simulink model "SF051A_SnsrOffsLrng"  (R2013b)
settings: Solver=FixedStepDiscrete  SolverMode=SingleTasking  StartTime=0.0  StopTime=1  FixedStep=0.002  RelTol=1e-3
undefined symbols (not defined in the file): ARCHGLBPRM_10MILLISEC_SEC_F32, ARCHGLBPRM_2MILLISEC_SEC_F32, ARCHGLBPRM_2PI_ULS_F32, ARCHGLBPRM_FLOATZEROTHD_ULS_F32, ARCHGLBPRM_PIOVER180_ULS_F32, CNV100MICROSECTOMILLISEC_MILLISECPERCNT_F32, CNV100MICROSECTOSEC_SECPERCNT_F32, COVRAMTRXNIT_ULS_F32, HWAUTHYTHD_ULS_F32, HWTQLRNGSTSLRND_CNT_U08, HWTQLRNGSTSNEGOFFS_CNT_U08, HWTQLRNGSTSNOTLRND_CNT_U08, HWTQLRNGSTSPOSOFFS_CNT_U08, HWTQLRNGSTSZEROOFFS_CNT_U08, HWTQLRNGTMRHILIM_SEC_F32, IDYMTRX_ULS_F32, IVS10MS_ULSPERSEC_F32, LRNGFILTICON_ULS_F32, NvmGetErrSts1, ONE_ULS_F32, SnsrOffsLrnd, SnsrOffsLrngFctEna, SnsrOffsLrngHwAgLrngDrvgDstThd, SnsrOffsLrngHwAgLrngEna, SnsrOffsLrngHwAgLrngHwVelThd, SnsrOffsLrngHwAgLrngSysTqThd, SnsrOffsLrngHwAgLrngSysTqThdMed, SnsrOffsLrngHwAgLrngSysTqThdTrustd, SnsrOffsLrngHwAgLrngSysTqThdWide, SnsrOffsLrngHwAgLrngTi, SnsrOffsLrngHwAgLrngVehSpdThd, SnsrOffsLrngHwAgLrngYawOffsDbnd, SnsrOffsLrngHwAgLrngYawRateThd, SnsrOffsLrngHwAgOffsLim, SnsrOffsLrngHwTqLrngEna, SnsrOffsLrngHwTqLrngEnaTiThd, SnsrOffsLrngHwTqLrngHwAgDbnd, SnsrOffsLrngHwTqLrngHwAgThd, SnsrOffsLrngHwTqLrngHwTqThd, SnsrOffsLrngHwTqLrngHwTqZeroOffsThd, SnsrOffsLrngHwTqLrngHwVelThd, SnsrOffsLrngHwTqLrngMeasTi, SnsrOffsLrngHwTqLrngMeasTiScar, SnsrOffsLrngHwTqLrngSampleImbThd1, SnsrOffsLrngHwTqLrngSampleImbThd2, SnsrOffsLrngHwTqLrngSampleThd1, SnsrOffsLrngHwTqLrngSampleThd2, SnsrOffsLrngHwTqLrngTiWghtCoeff, SnsrOffsLrngHwTqLrngVehSpdThd, SnsrOffsLrngHwTqOffsLim, SnsrOffsLrngSampleCntForHwTqLrngRst, SnsrOffsLrngTqInpDetnPwrEstimnThd, SnsrOffsLrngTqInpDetnSinGenrAmp, SnsrOffsLrngTqInpDetnSinGenrFrq, SnsrOffsLrngTqInpDetnStg1FilGain, SnsrOffsLrngTqInpDetnStg1WinSize, SnsrOffsLrngTqInpDetnStg2FilGainCen, SnsrOffsLrngTqInpDetnStg2FilGainDwn, SnsrOffsLrngTqInpDetnStg2FilGainUp, SnsrOffsLrngTqInpDetnStg2WinSize ... (+15)
libraries: Fil x34, FixdToFloat x17, FloatToFixd x16, NxtrLim x15, simulink x12, NxtrAbslt x12, NxtrNvM x8, NxtrMin x5, NxtrMath x3
(part 6 of 11)

== system SF051A_SnsrOffsLrng/SnsrOffsLrng/SnsrOffsLrngPer1/Measurements_Grabber/False ==
  Action Port : ActionPort  ActionType=then
  Constant : Constant  Value=false  OutDataTypeStr=boolean
      settings: AttributesFormatString=%<OutDataTypeStr>
  Constant2 : Constant  Value=ZERO_ULS_F32  OutDataTypeStr=single
      settings: AttributesFormatString=%<OutDataTypeStr>
  Subsystem5 : Subsystem  Description=|  mask(Copyright Information){none=on}
      | Copyright info block.                                               
      |                                                                     
      | Place copyright information at the top of every subsystem in design.
      mask prompts: none "No parameters"
      mask help: Place copyright information at the top of every subsystem in design.
      mask Display:
      | NxtrConf = 'Nexteer Confidential';
      | 
      | sys = bdroot; %handle for the current model ("system")
      | first = get_param(sys,'Created');
      | first = first(end-3:end);  %year is last four digits
      | 
      | last = get_param(sys,'LastModifiedDate');
      | if isempty(last)
      |     last = datestr(now,'yyyy');
      | else
      |     last = last(end-3:end);
      | end
      | 
      | if strcmp(first,last)
      |     fprintf('%s -- Copyright %s Nexteer',NxtrConf,first)
      | else
      |     fprintf('%s -- %s%s- %s Nexteer',NxtrConf,char(169),first,last)
      | end
  HwTqLrngLrngEna : Outport
  HwTq : Outport  Port=2
  HwAg : Outport  Port=3
  wires:
  Constant/1 -> HwTqLrngLrngEna/1
  Constant2/1 -> HwAg/1, HwTq/1

== system SF051A_SnsrOffsLrng/SnsrOffsLrng/SnsrOffsLrngPer1/Measurements_Grabber/GetTiSpan100MicroSec32bit ==
  note: Subtract original reference time
  note: seconds
  note: microseconds
  note: counts
  note: Wrap-to-zero
  note: 1 count = 100 uSec
  note: Get current system time
  note: GetTiSpan100MicroSec32bit
  note: Created Aug 18, 2015
      | Modified Oct 21, 2015
      | Modified Oct 30, 2015
      | Kevin Derry
  RefTmr : Inport
  CopyRight2 : Subsystem  Description=|  mask(Copyright Information){none=on}
      | Copyright info block.                                               
      |                                                                     
      | Place copyright information at the top of every subsystem in design.
      mask prompts: none "No parameters"
      mask help: Place copyright information at the top of every subsystem in design.
      mask Display:
      | NxtrConf = 'Nexteer Confidential';
      | 
      | sys = bdroot; %handle for the current model ("system")
      | first = get_param(sys,'Created');
      | if(isempty(first))
      |     first = datestr(now,'yyyy');
      | else
      |     first = first(end-3:end);  %year is last four digits
      | end
      | 
      | last = get_param(sys,'LastModifiedDate');
      | if isempty(last)
      |     last = datestr(now,'yyyy');
      | else
      |     last = last(end-3:end);
      | end
      | 
      | if strcmp(first,last)
      |     fprintf('%s -- Copyright %s Nexteer',NxtrConf,first)
      | else
      |     fprintf('%s -- %s%s- %s Nexteer',NxtrConf,char(169),first,last)
      | end
  Count per uSec : Constant  Value=0.01
  Data Store Read1 : DataStoreRead  DataStoreName=SimnTi
  Data Type Conversion2 : DataTypeConversion  OutDataTypeStr=uint32
  Divide1 : Product  Inputs=**
  Divide2 : Product  Inputs=*/
  If : If  NumInputs=2  IfExpression=u1 >= u2
  Max Counts : Constant  Value=2^32-1
  Merge : Merge
  No wrapping : Subsystem  TreatAsAtomicUnit=on
  Product2 : Product
  Product3 : Product
  Rounding : Rounding
  Subtract3 : Sum  Inputs=+-
  Wrapping : Subsystem  TreatAsAtomicUnit=on
  uSec per Sec : Constant  Value=1000000
  TiSpan : Outport
  wires:
  Wrapping/1(Out1) -> Merge/2
  No wrapping/1(Out1) -> Merge/1
  If/2 -> Wrapping/Action
  If/1 -> No wrapping/Action
  Product3/1 -> Subtract3/2
  Subtract3/1 -> Data Type Conversion2/1
  Rounding/1 -> Product3/1
  Divide2/1 -> Rounding/1
  Max Counts/1 -> Divide2/2, Product3/2
  Divide1/1 -> Divide2/1, Subtract3/1
  Product2/1 -> Divide1/1
  Data Store Read1/1 -> Product2/1
  Count per uSec/1 -> Divide1/2
  uSec per Sec/1 -> Product2/2
  Merge/1 -> TiSpan/1
  RefTmr/1 -> If/2, No wrapping/2(ref), Wrapping/2(ref)
  Data Type Conversion2/1 -> If/1, No wrapping/1(new), Wrapping/1(new)

== system SF051A_SnsrOffsLrng/SnsrOffsLrng/SnsrOffsLrngPer1/Measurements_Grabber/Subsystem5 ==

== system SF051A_SnsrOffsLrng/SnsrOffsLrng/SnsrOffsLrngPer1/Measurements_Grabber/True_UpdateNVMRam ==
  note: Set the Grabber Timer Reference back to current time.
  HwTq_in : Inport
  HwAg_in : Inport  Port=2
  Action Port : ActionPort  ActionType=else
  Constant : Constant  RequirementInfo={'linktype_rmi_doors' '0000babd (/E-STEER Core/SubSystem Specifications/Application Functions/SF051A Sensor Offset Learning)' '#SF051A_154' 'true' 'REQ:SF051A_154' '' } %GIDa_348884a7_199b_420e_8b8f_aec7d8a42fd4  Value=true  OutDataTypeStr=boolean
      settings: AttributesFormatString=%<OutDataTypeStr>
  Data Store Write : DataStoreWrite  DataStoreName=HwTqLrngMeasTmrRef
  FloatToFixd_s16_f32 : FloatToFixd/FloatToFixd_s16_f32  Param1=4
  GetRefTmr100MicroSec32bit : Subsystem
  NvmRam : DataStoreWrite  RequirementInfo={'linktype_rmi_doors' '0000babd (/E-STEER Core/SubSystem Specifications/Application Functions/SF051A Sensor Offset Learning)' '#SF051A_153' 'true' 'REQ:SF051A_153' '' } %GIDa_33126d3e_f2c5_434b_b28a_2b62a4ba3060  DataStoreName=SnsrOffsLrnd  DataStoreElements=SnsrOffsLrnd.HwTqLrngHwAgRef
  Subsystem5 : Subsystem  Description=|  mask(Copyright Information){none=on}
      | Copyright info block.                                               
      |                                                                     
      | Place copyright information at the top of every subsystem in design.
      mask prompts: none "No parameters"
      mask help: Place copyright information at the top of every subsystem in design.
      mask Display:
      | NxtrConf = 'Nexteer Confidential';
      | 
      | sys = bdroot; %handle for the current model ("system")
      | first = get_param(sys,'Created');
      | first = first(end-3:end);  %year is last four digits
      | 
      | last = get_param(sys,'LastModifiedDate');
      | if isempty(last)
      |     last = datestr(now,'yyyy');
      | else
      |     last = last(end-3:end);
      | end
      | 
      | if strcmp(first,last)
      |     fprintf('%s -- Copyright %s Nexteer',NxtrConf,first)
      | else
      |     fprintf('%s -- %s%s- %s Nexteer',NxtrConf,char(169),first,last)
      | end
  HwTqLrngLrngEna : Outport  RequirementInfo={'linktype_rmi_doors' '0000babd (/E-STEER Core/SubSystem Specifications/Application Functions/SF051A Sensor Offset Learning)' '#SF051A_154' 'true' 'REQ:SF051A_154' '' } %GIDa_4152f285_7238_40df_a9ce_ba8c043104c1
  HwTq : Outport  Port=2
  HwAg : Outport  Port=3
  wires:
  Constant/1 -> HwTqLrngLrngEna/1
  HwAg_in/1 -> FloatToFixd_s16_f32/1, HwAg/1
  HwTq_in/1 -> HwTq/1
  GetRefTmr100MicroSec32bit/1(RefTmr) -> Data Store Write/1
  FloatToFixd_s16_f32/1 -> NvmRam/1

== system SF051A_SnsrOffsLrng/SnsrOffsLrng/SnsrOffsLrngPer1/SetFalse/Subsystem1 ==

== system SF051A_SnsrOffsLrng/SnsrOffsLrng/SnsrOffsLrngPer1/Zero_GrabberTimer/GetRefTmr100MicroSec32bit ==
  note: 1 count = 100 uSec
  note: seconds
  note: microseconds
  note: counts
  note: Wrap-to-zero
  note: GetRefTmr100MicroSec32bit
  note: Created Aug 18, 2015
      | Modified Oct 21, 2015
      | Modified Oct 30, 2015
      | Kevin Derry
  CopyRight2 : Subsystem  Description=|  mask(Copyright Information){none=on}
      | Copyright info block.                                               
      |                                                                     
      | Place copyright information at the top of every subsystem in design.
      mask prompts: none "No parameters"
      mask help: Place copyright information at the top of every subsystem in design.
      mask Display:
      | NxtrConf = 'Nexteer Confidential';
      | 
      | sys = bdroot; %handle for the current model ("system")
      | first = get_param(sys,'Created');
      | if(isempty(first))
      |     first = datestr(now,'yyyy');
      | else
      |     first = first(end-3:end);  %year is last four digits
      | end
      | 
      | last = get_param(sys,'LastModifiedDate');
      | if isempty(last)
      |     last = datestr(now,'yyyy');
      | else
      |     last = last(end-3:end);
      | end
      | 
      | if strcmp(first,last)
      |     fprintf('%s -- Copyright %s Nexteer',NxtrConf,first)
      | else
      |     fprintf('%s -- %s%s- %s Nexteer',NxtrConf,char(169),first,last)
      | end
  Count per uSec : Constant  Value=0.01
  Data Store Read1 : DataStoreRead  DataStoreName=SimnTi
  Data Type Conversion1 : DataTypeConversion  OutDataTypeStr=uint32
  Divide1 : Product  Inputs=**
  Divide2 : Product  Inputs=*/
  Max Counts : Constant  Value=2^32-1
  Product1 : Product
  Product2 : Product
  Rounding : Rounding
  Subtract1 : Sum  Inputs=+-
  uSec per Sec : Constant  Value=1000000
  RefTmr : Outport
  wires:
  Product2/1 -> Subtract1/2
  Subtract1/1 -> Data Type Conversion1/1
  Rounding/1 -> Product2/1
  Divide2/1 -> Rounding/1
  Max Counts/1 -> Divide2/2, Product2/2
  Divide1/1 -> Divide2/1, Subtract1/1
  Product1/1 -> Divide1/1
  Count per uSec/1 -> Divide1/2
  uSec per Sec/1 -> Product1/2
  Data Type Conversion1/1 -> RefTmr/1
  Data Store Read1/1 -> Product1/1

== system SF051A_SnsrOffsLrng/SnsrOffsLrng/SnsrOffsLrngPer1/Zero_GrabberTimer/Subsystem5 ==

== system SF051A_SnsrOffsLrng/SnsrOffsLrng/SnsrOffsLrngPer2/Do nothing/Subsystem5 ==

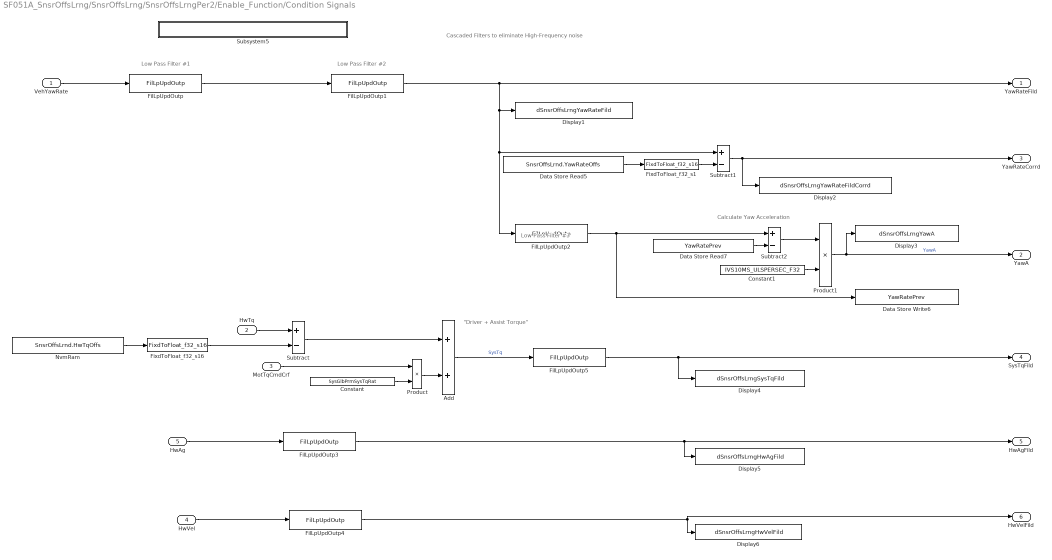
== system SF051A_SnsrOffsLrng/SnsrOffsLrng/SnsrOffsLrngPer2/Enable_Function/Condition Signals ==
  note: Calculate Yaw Acceleration
  note: Low Pass Filter #1
  note: Cascaded Filters to eliminate High-Frequency noise
  note: Low Pass Filter #2
  note: "Driver + Assist Torque"
  note: Low Pass Filter #3
  VehYawRate : Inport
  HwTq : Inport  RequirementInfo={'linktype_rmi_doors' '0000babd (/E-STEER Core/SubSystem Specifications/Application Functions/SF051A Sensor Offset Learning)' '#SF051A_88' 'true' 'REQ:SF051A_88' '' } %GIDa_cb0b5578_d931_4b15_8fb5_23406b09174e  Port=2
  MotTqCmdCrf : Inport  RequirementInfo={'linktype_rmi_doors' '0000babd (/E-STEER Core/SubSystem Specifications/Application Functions/SF051A Sensor Offset Learning)' '#SF051A_87' 'true' 'REQ:SF051A_87' '' } %GIDa_6e162c2c_edb1_407c_9856_d4fb5c13668b  Port=3
  HwVel : Inport  Port=4
  HwAg : Inport  Port=5
  Add : Sum  RequirementInfo={'linktype_rmi_doors' '0000babd (/E-STEER Core/SubSystem Specifications/Application Functions/SF051A Sensor Offset Learning)' '#SF051A_87' 'true' 'REQ:SF051A_87' '' } %GIDa_ae37b931_f532_4a31_8fdb_8a3b99cf0b70
  Constant : Constant  RequirementInfo={'linktype_rmi_doors' '0000babd (/E-STEER Core/SubSystem Specifications/Application Functions/SF051A Sensor Offset Learning)' '#SF051A_87' 'true' 'REQ:SF051A_87' '' } %GIDa_19f7d8cf_06b3_41bf_b52b_b35be25960ea  Value=SysGlbPrmSysTqRat
  Constant1 : Constant  RequirementInfo={'linktype_rmi_doors' '0000babd (/E-STEER Core/SubSystem Specifications/Application Functions/SF051A Sensor Offset Learning)' '#SF051A_89' 'true' 'REQ:SF051A_89' '' } %GIDa_346656a3_816f_4164_b776_9fdc6d4ed815  Value=IVS10MS_ULSPERSEC_F32  OutDataTypeStr=single
  Data Store Read5 : DataStoreRead  RequirementInfo={'linktype_rmi_doors' '0000babd (/E-STEER Core/SubSystem Specifications/Application Functions/SF051A Sensor Offset Learning)' '#SF051A_29' 'true' 'REQ:SF051A_29' '' } %GIDa_fe5ea230_6dba_49b3_a98a_1e7dfb304a5e  DataStoreName=SnsrOffsLrnd  DataStoreElements=SnsrOffsLrnd.YawRateOffs
  Data Store Read7 : DataStoreRead  RequirementInfo={'linktype_rmi_doors' '0000babd (/E-STEER Core/SubSystem Specifications/Application Functions/SF051A Sensor Offset Learning)' '#SF051A_89' 'true' 'REQ:SF051A_89' '' } %GIDa_851ad77d_6e53_4d8f_a6a0_8bfa0b715fb5  Priority=1  DataStoreName=YawRatePrev
      settings: AttributesFormatString=priority: %<Priority>
  Data Store Write6 : DataStoreWrite  Priority=2  DataStoreName=YawRatePrev
      settings: AttributesFormatString=priority: %<Priority>
  Display1 : DataStoreWrite  DataStoreName=dSnsrOffsLrngYawRateFild
  Display2 : DataStoreWrite  DataStoreName=dSnsrOffsLrngYawRateFildCorrd
  Display3 : DataStoreWrite  DataStoreName=dSnsrOffsLrngYawA
  Display4 : DataStoreWrite  DataStoreName=dSnsrOffsLrngSysTqFild
  Display5 : DataStoreWrite  DataStoreName=dSnsrOffsLrngHwAgFild
  Display6 : DataStoreWrite  DataStoreName=dSnsrOffsLrngHwVelFild
  FilLpUpdOutp : Fil/FilLpUpdOutp  RequirementInfo={'linktype_rmi_doors' '0000babd (/E-STEER Core/SubSystem Specifications/Application Functions/SF051A Sensor Offset Learning)' '#SF051A_28' 'true' 'REQ:SF051A_28' '' } %GIDa_8a84e711_3ffa_4571_bf4b_e7f85249d077  StVar=YawCdngFil1
      settings: AttributesFormatString=StVar: %<StVar>
  FilLpUpdOutp1 : Fil/FilLpUpdOutp  RequirementInfo={'linktype_rmi_doors' '0000babd (/E-STEER Core/SubSystem Specifications/Application Functions/SF051A Sensor Offset Learning)' '#SF051A_28' 'true' 'REQ:SF051A_28' '' } %GIDa_c79bec69_8b23_4153_99a8_6f46e3270235  StVar=YawCdngFil2
      settings: AttributesFormatString=StVar: %<StVar>
  FilLpUpdOutp2 : Fil/FilLpUpdOutp  StVar=YawACdngFil
      settings: AttributesFormatString=StVar: %<StVar>
  FilLpUpdOutp3 : Fil/FilLpUpdOutp  RequirementInfo={'linktype_rmi_doors' '0000babd (/E-STEER Core/SubSystem Specifications/Application Functions/SF051A Sensor Offset Learning)' '#SF051A_28' 'true' 'REQ:SF051A_28' '' } %GIDa_cea2d234_d78b_493c_8f76_fa1ba10d1cf3  StVar=HwAgCdngFil
      settings: AttributesFormatString=StVar: %<StVar>
  FilLpUpdOutp4 : Fil/FilLpUpdOutp  RequirementInfo={'linktype_rmi_doors' '0000babd (/E-STEER Core/SubSystem Specifications/Application Functions/SF051A Sensor Offset Learning)' '#SF051A_28' 'true' 'REQ:SF051A_28' '' } %GIDa_c5648a7c_47c7_487c_beaa_905359562805  StVar=HwVelCdngFil
      settings: AttributesFormatString=StVar: %<StVar>
  FilLpUpdOutp5 : Fil/FilLpUpdOutp  RequirementInfo={'linktype_rmi_doors' '0000babd (/E-STEER Core/SubSystem Specifications/Application Functions/SF051A Sensor Offset Learning)' '#SF051A_28' 'true' 'REQ:SF051A_28' '' } %GIDa_a435df6e_5d26_4266_822f_3dfbe8640535  StVar=SysTqCdngFil
      settings: AttributesFormatString=StVar: %<StVar>
  FixdToFloat_f32_s1 : FixdToFloat/FixdToFloat_f32_s16  RequirementInfo={'linktype_rmi_doors' '0000babd (/E-STEER Core/SubSystem Specifications/Application Functions/SF051A Sensor Offset Learning)' '#SF051A_29' 'true' 'REQ:SF051A_29' '' } %GIDa_3d73e24e_fd42_443d_a6ec_262aa8637762  Param1=9
  FixdToFloat_f32_s16 : FixdToFloat/FixdToFloat_f32_s16  RequirementInfo={'linktype_rmi_doors' '0000babd (/E-STEER Core/SubSystem Specifications/Application Functions/SF051A Sensor Offset Learning)' '#SF051A_88' 'true' 'REQ:SF051A_88' '' } %GIDa_748ccc23_09d4_473b_a4ee_8bbea57db921  Param1=12
  NvmRam : DataStoreRead  RequirementInfo={'linktype_rmi_doors' '0000babd (/E-STEER Core/SubSystem Specifications/Application Functions/SF051A Sensor Offset Learning)' '#SF051A_88' 'true' 'REQ:SF051A_88' '' } %GIDa_4121cf44_6622_4a9b_8e6c_74768dd324f4  DataStoreName=SnsrOffsLrnd  DataStoreElements=SnsrOffsLrnd.HwTqOffs
  Product : Product  RequirementInfo={'linktype_rmi_doors' '0000babd (/E-STEER Core/SubSystem Specifications/Application Functions/SF051A Sensor Offset Learning)' '#SF051A_87' 'true' 'REQ:SF051A_87' '' } %GIDa_e0b80c88_6c4b_4ba5_b309_b8f72dd11838
  Product1 : Product  RequirementInfo={'linktype_rmi_doors' '0000babd (/E-STEER Core/SubSystem Specifications/Application Functions/SF051A Sensor Offset Learning)' '#SF051A_89' 'true' 'REQ:SF051A_89' '' } %GIDa_0d782124_913b_4f0a_847b_c237fe5371b9
  Subsystem5 : Subsystem  Description=|  mask(Copyright Information){none=on}
      | Copyright info block.                                               
      |                                                                     
      | Place copyright information at the top of every subsystem in design.
      mask prompts: none "No parameters"
      mask help: Place copyright information at the top of every subsystem in design.
      mask Display:
      | NxtrConf = 'Nexteer Confidential';
      | 
      | sys = bdroot; %handle for the current model ("system")
      | first = get_param(sys,'Created');
      | first = first(end-3:end);  %year is last four digits
      | 
      | last = get_param(sys,'LastModifiedDate');
      | if isempty(last)
      |     last = datestr(now,'yyyy');
      | else
      |     last = last(end-3:end);
      | end
      | 
      | if strcmp(first,last)
      |     fprintf('%s -- Copyright %s Nexteer',NxtrConf,first)
      | else
      |     fprintf('%s -- %s%s- %s Nexteer',NxtrConf,char(169),first,last)
      | end
  Subtract : Sum  RequirementInfo={'linktype_rmi_doors' '0000babd (/E-STEER Core/SubSystem Specifications/Application Functions/SF051A Sensor Offset Learning)' '#SF051A_88' 'true' 'REQ:SF051A_88' '' ; 'linktype_rmi_doors' '0000babd (/E-STEER Core/SubSystem Specifications/Application Functions/SF051A Sensor Offset Learning)' '#SF051A_87' 'true' 'REQ:SF051A_87' '' } %GIDa_99fe81ca_b737_406d_903a_82e012cba0fe  Inputs=+-
  Subtract1 : Sum  RequirementInfo={'linktype_rmi_doors' '0000babd (/E-STEER Core/SubSystem Specifications/Application Functions/SF051A Sensor Offset Learning)' '#SF051A_29' 'true' 'REQ:SF051A_29' '' } %GIDa_5e83f16f_2d18_4316_802f_cef8993711a6  Inputs=+-
  Subtract2 : Sum  RequirementInfo={'linktype_rmi_doors' '0000babd (/E-STEER Core/SubSystem Specifications/Application Functions/SF051A Sensor Offset Learning)' '#SF051A_89' 'true' 'REQ:SF051A_89' '' } %GIDa_c77efd6a_eb15_4122_9f5d_3e3beff93d42  Inputs=+-
  YawRateFild : Outport
  YawA : Outport  Port=2
  YawRateCorrd : Outport  Port=3  OutDataTypeStr=single
  SysTqFild : Outport  Port=4
  HwAgFild : Outport  Port=5
  HwVelFild : Outport  Port=6
  wires:
  VehYawRate/1 -> FilLpUpdOutp/1
  FilLpUpdOutp1/1 -> Display1/1, FilLpUpdOutp2/1, Subtract1/1, YawRateFild/1
  HwTq/1 -> Subtract/1
  FixdToFloat_f32_s16/1 -> Subtract/2
  Subtract/1 -> Add/1
  MotTqCmdCrf/1 -> Product/1
  Product/1 -> Add/2
  Constant/1 -> Product/2
  HwAg/1 -> FilLpUpdOutp3/1
  FilLpUpdOutp3/1 -> Display5/1, HwAgFild/1
  Add/1 -> FilLpUpdOutp5/1  "SysTq"
  HwVel/1 -> FilLpUpdOutp4/1
  FilLpUpdOutp4/1 -> HwVelFild/1, Display6/1
  Data Store Read5/1 -> FixdToFloat_f32_s1/1
  Subtract1/1 -> Display2/1, YawRateCorrd/1
  FilLpUpdOutp2/1 -> Subtract2/1, Data Store Write6/1
  Subtract2/1 -> Product1/1
  Constant1/1 -> Product1/2
  Product1/1 -> Display3/1, YawA/1  "YawA"
  Data Store Read7/1 -> Subtract2/2
  NvmRam/1 -> FixdToFloat_f32_s16/1
  FixdToFloat_f32_s1/1 -> Subtract1/2
  FilLpUpdOutp/1 -> FilLpUpdOutp1/1
  FilLpUpdOutp5/1 -> Display4/1, SysTqFild/1

== system SF051A_SnsrOffsLrng/SnsrOffsLrng/SnsrOffsLrngPer2/Enable_Function/POC ==
  note: Reset HwTq learning if requested by Hierarch Manager routine.
  note: Learn HwAg Offset if contitions are appropriate
  YawRateCorrd : Inport  RequirementInfo={'linktype_rmi_doors' '0000babd (/E-STEER Core/SubSystem Specifications/Application Functions/SF051A Sensor Offset Learning)' '#SF051A_131' 'true' 'REQ:SF051A_131' '' } %GIDa_2241a612_69c9_42e1_bc9a_8143374c6a10
  SysTqFild : Inport  RequirementInfo={'linktype_rmi_doors' '0000babd (/E-STEER Core/SubSystem Specifications/Application Functions/SF051A Sensor Offset Learning)' '#SF051A_130' 'true' 'REQ:SF051A_130' '' } %GIDa_8ac64dc8_efd4_4fea_8be1_3530061f71ef  Port=2
  HwAgFild : Inport  RequirementInfo={'linktype_rmi_doors' '0000babd (/E-STEER Core/SubSystem Specifications/Application Functions/SF051A Sensor Offset Learning)' '#SF051A_132' 'true' 'REQ:SF051A_132' '' } %GIDa_f9032355_6dd8_4cb3_b45a_f22c4cf0875b  Port=3
  HwVelFild : Inport  RequirementInfo={'linktype_rmi_doors' '0000babd (/E-STEER Core/SubSystem Specifications/Application Functions/SF051A Sensor Offset Learning)' '#SF051A_129' 'true' 'REQ:SF051A_129' '' } %GIDa_c6634e4e_7c1b_460a_a499_07b7e4fc4f6e  Port=4
  HwAgLrngEna : Inport  Port=5  OutDataTypeStr=boolean
  VehSpd : Inport  RequirementInfo={'linktype_rmi_doors' '0000babd (/E-STEER Core/SubSystem Specifications/Application Functions/SF051A Sensor Offset Learning)' '#SF051A_133' 'true' 'REQ:SF051A_133' '' } %GIDa_d75244df_0bb9_4d68_80fb_b65b4be69888  Port=6
  HwTqLrngSts : Inport  RequirementInfo={'linktype_rmi_doors' '0000babd (/E-STEER Core/SubSystem Specifications/Application Functions/SF051A Sensor Offset Learning)' '#SF051A_128' 'true' 'REQ:SF051A_128' '' } %GIDa_340de515_3a73_4d29_9413_69b747b6f805  Port=7
  HwAgLrngRst : Inport  Port=8
  Do nothing : Subsystem  TreatAsAtomicUnit=on
  Do nothing1 : Subsystem  TreatAsAtomicUnit=on
  If : If  RequirementInfo={'linktype_rmi_doors' '0000babd (/E-STEER Core/SubSystem Specifications/Application Functions/SF051A Sensor Offset Learning)' '#SF051A_124' 'true' 'REQ:SF051A_124' '' } %GIDa_5a1c07af_5997_48cd_9c05_bf217e97f002  NumInputs=2  IfExpression=u1 & u2
  If1 : If  IfExpression=u1
  Learn : Subsystem  RequirementInfo={'linktype_rmi_doors' '0000babd (/E-STEER Core/SubSystem Specifications/Application Functions/SF051A Sensor Offset Learning)' '#SF051A_127' 'true' 'REQ:SF051A_127' '' } %GIDa_6eb60759_6337_4052_a701_a1794125d7b8  TreatAsAtomicUnit=on
  Learning Conditions : Subsystem  RequirementInfo={'linktype_rmi_doors' '0000babd (/E-STEER Core/SubSystem Specifications/Application Functions/SF051A Sensor Offset Learning)' '#SF051A_126' 'true' 'REQ:SF051A_126' '' } %GIDa_668521da_dfcc_45f6_9303_a91806d72581
  Reset_HwAg_Learning : Subsystem  TreatAsAtomicUnit=on
  Subsystem5 : Subsystem  Description=|  mask(Copyright Information){none=on}
      | Copyright info block.                                               
      |                                                                     
      | Place copyright information at the top of every subsystem in design.
      mask prompts: none "No parameters"
      mask help: Place copyright information at the top of every subsystem in design.
      mask Display:
      | NxtrConf = 'Nexteer Confidential';
      | 
      | sys = bdroot; %handle for the current model ("system")
      | first = get_param(sys,'Created');
      | first = first(end-3:end);  %year is last four digits
      | 
      | last = get_param(sys,'LastModifiedDate');
      | if isempty(last)
      |     last = datestr(now,'yyyy');
      | else
      |     last = last(end-3:end);
      | end
      | 
      | if strcmp(first,last)
      |     fprintf('%s -- Copyright %s Nexteer',NxtrConf,first)
      | else
      |     fprintf('%s -- %s%s- %s Nexteer',NxtrConf,char(169),first,last)
      | end
  wires:
  VehSpd/1 -> Learning Conditions/1(VehSpd)
  HwAgFild/1 -> Learn/1(HwAgFild)
  HwVelFild/1 -> Learning Conditions/2(HwVelFild)
  YawRateCorrd/1 -> Learning Conditions/3(YawRateCorrd)
  HwAgLrngEna/1 -> If/1  "HwAgLrngEna"
  HwTqLrngSts/1 -> Learn/3(HwTqLrngSts)
  Learning Conditions/1(LrngCdnVld) -> If/2
  If/1 -> Learn/Action
  SysTqFild/1 -> Learn/2(SysTrqFild), Learning Conditions/4(SysTqFild)
  If/2 -> Do nothing/Action
  HwAgLrngRst/1 -> If1/1
  If1/1 -> Reset_HwAg_Learning/Action
  If1/2 -> Do nothing1/Action

== system SF051A_SnsrOffsLrng/SnsrOffsLrng/SnsrOffsLrngPer2/Enable_Function/SOaC_HierarchyManager ==
  YawRateOffsFrsh : Inport
  HwAgAuthy : Inport  Port=2
  VehSpdVld : Inport  Port=3
  VehYawRateVld : Inport  Port=4
  Constant : Constant  Value=HWAUTHYTHD_ULS_F32
  Logical Operator : Logic  AllPortsSameDT=off  OutDataTypeStr=boolean
  POCEnabler : Subsystem
  POCResetLogic : Subsystem
  Relational Operator : RelationalOperator  OutDataTypeStr=boolean
  Subsystem5 : Subsystem  Description=|  mask(Copyright Information){none=on}
      | Copyright info block.                                               
      |                                                                     
      | Place copyright information at the top of every subsystem in design.
      mask prompts: none "No parameters"
      mask help: Place copyright information at the top of every subsystem in design.
      mask Display:
      | NxtrConf = 'Nexteer Confidential';
      | 
      | sys = bdroot; %handle for the current model ("system")
      | first = get_param(sys,'Created');
      | first = first(end-3:end);  %year is last four digits
      | 
      | last = get_param(sys,'LastModifiedDate');
      | if isempty(last)
      |     last = datestr(now,'yyyy');
      | else
      |     last = last(end-3:end);
      | end
      | 
      | if strcmp(first,last)
      |     fprintf('%s -- Copyright %s Nexteer',NxtrConf,first)
      | else
      |     fprintf('%s -- %s%s- %s Nexteer',NxtrConf,char(169),first,last)
      | end
  YOCEnabler : Subsystem
  YawRateLrngEna : Outport
  HwAgLrngEna : Outport  Port=2
  HwAgLrngRst : Outport  Port=3
  wires:
  POCResetLogic/1(HwAgLrngRst) -> HwAgLrngRst/1
  POCEnabler/1(HwAgLrngEna) -> HwAgLrngEna/1
  YOCEnabler/1(YawRateLrngEna) -> YawRateLrngEna/1
  Relational Operator/1 -> Logical Operator/1
  VehSpdVld/1 -> Logical Operator/2
  VehYawRateVld/1 -> YOCEnabler/2(VehYawRateVld), POCEnabler/2(VehYawRateVld)
  HwAgAuthy/1 -> Relational Operator/1
  Logical Operator/1 -> YOCEnabler/1(CmnSigVld), [CmnSigVld]  "CmnSigVld"
  [CmnSigVld] -> POCEnabler/1(CmnSigVld)
  YawRateOffsFrsh/1 -> POCEnabler/3(YawRateOffsFrsh)
  Constant/1 -> Relational Operator/2

== system SF051A_SnsrOffsLrng/SnsrOffsLrng/SnsrOffsLrngPer2/Enable_Function/Subsystem5 ==

== system SF051A_SnsrOffsLrng/SnsrOffsLrng/SnsrOffsLrngPer2/Enable_Function/YOC ==
  note: Limit changed to a Min block. Code might not be affected.
  note: Every execution loop of Periodic 2, the yaw rate freshness timer increments.  Using a loop counter instead of client calls
      | because the elapsed time is "frozen" across ignition cycles.  The counter is reset to zero when learning occurs.
  note: When vehicle conditions are right and all bus signals are valid, begin or continue learning.
  YawRateLrngEna : Inport
  YawRateFild : Inport  RequirementInfo={'linktype_rmi_doors' '0000babd (/E-STEER Core/SubSystem Specifications/Application Functions/SF051A Sensor Offset Learning)' '#SF051A_100' 'true' 'REQ:SF051A_100' '' } %GIDa_4788fb8c_6bdd_419e_be01_c723b642e277  Port=2
  YawA : Inport  RequirementInfo={'linktype_rmi_doors' '0000babd (/E-STEER Core/SubSystem Specifications/Application Functions/SF051A Sensor Offset Learning)' '#SF051A_99' 'true' 'REQ:SF051A_99' '' } %GIDa_1132fb7b_54bf_40b1_acf5_f9054bb6ad26  Port=3
  VehSpd : Inport  RequirementInfo={'linktype_rmi_doors' '0000babd (/E-STEER Core/SubSystem Specifications/Application Functions/SF051A Sensor Offset Learning)' '#SF051A_102' 'true' 'REQ:SF051A_102' '' } %GIDa_5315707f_4311_4e1a_9598_78d874dd3bdb  Port=4
  HwAg : Inport  RequirementInfo={'linktype_rmi_doors' '0000babd (/E-STEER Core/SubSystem Specifications/Application Functions/SF051A Sensor Offset Learning)' '#SF051A_101' 'true' 'REQ:SF051A_101' '' } %GIDa_72eb9de4_dd58_44cc_88ca_111522a15ca4  Port=5
  Add : Sum
  Constant : Constant  RequirementInfo={'linktype_rmi_doors' '0000babd (/E-STEER Core/SubSystem Specifications/Application Functions/SF051A Sensor Offset Learning)' '#SF051A_111' 'true' 'REQ:SF051A_111' '' ; 'linktype_rmi_doors' '0000babd (/E-STEER Core/SubSystem Specifications/Application Functions/SF051A Sensor Offset Learning)' '#SF051A_242' 'true' 'REQ:SF051A_242' '' } %GIDa_883fb207_2bdb_43f4_8fbf_3d3c8800e308  Value=SnsrOffsLrngYawOffsFrshTiThd  OutDataTypeStr=single
  Constant1 : Constant  Value=TISTEP10MS_MINS_F32  OutDataTypeStr=single
  Constant2 : Constant  Value=SnsrOffsLrngYawOffsFrshTiThd  OutDataTypeStr=single
  Data Store Read : DataStoreRead  DataStoreName=SnsrOffsLrnd  DataStoreElements=SnsrOffsLrnd.YawRateElpdTi
  Data Store Write : DataStoreWrite  DataStoreName=SnsrOffsLrnd  DataStoreElements=SnsrOffsLrnd.YawRateElpdTi
  Data Store Write1 : DataStoreWrite  RequirementInfo={'linktype_rmi_doors' '0000babd (/E-STEER Core/SubSystem Specifications/Application Functions/SF051A Sensor Offset Learning)' '#SF051A_112' 'true' 'REQ:SF051A_112' '' } %GIDa_1386d18f_d052_4548_b025_86f8f1b54bd3  DataStoreName=VehYawRateOffsFrsh
  Do nothing : Subsystem  TreatAsAtomicUnit=on
  If : If  RequirementInfo={'linktype_rmi_doors' '0000babd (/E-STEER Core/SubSystem Specifications/Application Functions/SF051A Sensor Offset Learning)' '#SF051A_95' 'true' 'REQ:SF051A_95' '' } %GIDa_5a0d1c96_ac6c_4e69_b879_396e00cbc286  NumInputs=2  IfExpression=u1 & u2
  Learn : Subsystem  RequirementInfo={'linktype_rmi_doors' '0000babd (/E-STEER Core/SubSystem Specifications/Application Functions/SF051A Sensor Offset Learning)' '#SF051A_94' 'true' 'REQ:SF051A_94' '' } %GIDa_548ddfb5_a741_4714_aec1_02ee3ee42dbb  TreatAsAtomicUnit=on
  Learning Conditions : Subsystem  RequirementInfo={'linktype_rmi_doors' '0000babd (/E-STEER Core/SubSystem Specifications/Application Functions/SF051A Sensor Offset Learning)' '#SF051A_97' 'true' 'REQ:SF051A_97' '' ; 'linktype_rmi_doors' '0000babd (/E-STEER Core/SubSystem Specifications/Application Functions/SF051A Sensor Offset Learning)' '#SF051A_96' 'true' 'REQ:SF051A_96' '' } %GIDa_890fa9a9_e67d_4d09_8fef_362b51c9d8ff
  Min_f32 : NxtrMin/Min_f32  SFunctionSpec=single y1 = Min_f32(single u1, single u2)
      settings: AttributesFormatString=%<Name>
  Relational Operator : RelationalOperator  RequirementInfo={'linktype_rmi_doors' '0000babd (/E-STEER Core/SubSystem Specifications/Application Functions/SF051A Sensor Offset Learning)' '#SF051A_111' 'true' 'REQ:SF051A_111' '' ; 'linktype_rmi_doors' '0000babd (/E-STEER Core/SubSystem Specifications/Application Functions/SF051A Sensor Offset Learning)' '#SF051A_242' 'true' 'REQ:SF051A_242' '' } %GIDa_100189d6_4f90_49af_8752_2852919b8786  Operator=<=  OutDataTypeStr=boolean
  Subsystem5 : Subsystem  Description=|  mask(Copyright Information){none=on}
      | Copyright info block.                                               
      |                                                                     
      | Place copyright information at the top of every subsystem in design.
      mask prompts: none "No parameters"
      mask help: Place copyright information at the top of every subsystem in design.
      mask Display:
      | NxtrConf = 'Nexteer Confidential';
      | 
      | sys = bdroot; %handle for the current model ("system")
      | first = get_param(sys,'Created');
      | first = first(end-3:end);  %year is last four digits
      | 
      | last = get_param(sys,'LastModifiedDate');
      | if isempty(last)
      |     last = datestr(now,'yyyy');
      | else
      |     last = last(end-3:end);
      | end
      | 
      | if strcmp(first,last)
      |     fprintf('%s -- Copyright %s Nexteer',NxtrConf,first)
      | else
      |     fprintf('%s -- %s%s- %s Nexteer',NxtrConf,char(169),first,last)
      | end
  wires:
  YawRateFild/1 -> Learning Conditions/4(YawRateFild), Learn/1(YawRate)
  Learning Conditions/1(LrngCdnVld) -> If/2
  YawRateLrngEna/1 -> If/1
  VehSpd/1 -> Learning Conditions/1(VehSpd)
  HwAg/1 -> Learning Conditions/2(HwAg)
  If/1 -> Learn/Action
  Constant/1 -> Relational Operator/2
  Data Store Read/1 -> Add/1
  Constant1/1 -> Add/2
  Add/1 -> Relational Operator/1, Min_f32/1  "ElpsdTi"
  Min_f32/1 -> Data Store Write/1
  YawA/1 -> Learning Conditions/3(YawA)
  If/2 -> Do nothing/Action
  Relational Operator/1 -> Data Store Write1/1
  Constant2/1 -> Min_f32/2

== system SF051A_SnsrOffsLrng/SnsrOffsLrng/SetHwTqOffs/Reset Learning/GetRefTmr100MicroSec32bit/CopyRight2 ==

== system SF051A_SnsrOffsLrng/SnsrOffsLrng/SnsrOffsLrngInit1/NVM Management/Data Invalid/Subsystem5 ==

== system SF051A_SnsrOffsLrng/SnsrOffsLrng/SnsrOffsLrngInit1/NVM Management/Data Valid/Subsystem5 ==

== system SF051A_SnsrOffsLrng/SnsrOffsLrng/SnsrOffsLrngInit1/NVM Management/Not Enabled/Subsystem5 ==

== system SF051A_SnsrOffsLrng/SnsrOffsLrng/SnsrOffsLrngPer1/EnableLearning/Default_TqInpDetn/Subsystem5 ==

== system SF051A_SnsrOffsLrng/SnsrOffsLrng/SnsrOffsLrngPer1/EnableLearning/EnablingConditions/CheckLastMeasHwPos ==
  HwAg : Inport
  Abslt_f32_f32 : NxtrAbslt/Abslt_f32_f32  SFunctionSpec=single y1 = Abslt_f32_f32(single u1)
      settings: AttributesFormatString=%<Name>
  Constant : Constant  Value=SnsrOffsLrngHwTqLrngHwAgDbnd
  Data Store Read : DataStoreRead  DataStoreName=SnsrOffsLrnd  DataStoreElements=SnsrOffsLrnd.HwTqLrngHwAgRef
  FalseOut_KeepRef : Subsystem  TreatAsAtomicUnit=on
  FixdToFloat_f32_s16 : FixdToFloat/FixdToFloat_f32_s16  Param1=4
  If : If  IfExpression=u1
  Merge : Merge
  Relational Operator : RelationalOperator  OutDataTypeStr=boolean
  Subsystem5 : Subsystem  Description=|  mask(Copyright Information){none=on}
      | Copyright info block.                                               
      |                                                                     
      | Place copyright information at the top of every subsystem in design.
      mask prompts: none "No parameters"
      mask help: Place copyright information at the top of every subsystem in design.
      mask Display:
      | NxtrConf = 'Nexteer Confidential';
      | 
      | sys = bdroot; %handle for the current model ("system")
      | first = get_param(sys,'Created');
      | first = first(end-3:end);  %year is last four digits
      | 
      | last = get_param(sys,'LastModifiedDate');
      | if isempty(last)
      |     last = datestr(now,'yyyy');
      | else
      |     last = last(end-3:end);
      | end
      | 
      | if strcmp(first,last)
      |     fprintf('%s -- Copyright %s Nexteer',NxtrConf,first)
      | else
      |     fprintf('%s -- %s%s- %s Nexteer',NxtrConf,char(169),first,last)
      | end
  Subtract : Sum  Inputs=+-
  TrueOut_ResetRef : Subsystem  TreatAsAtomicUnit=on
  HwAgMoved : Outport
  wires:
  Relational Operator/1 -> If/1
  Constant/1 -> Relational Operator/2
  Data Store Read/1 -> FixdToFloat_f32_s16/1
  HwAg/1 -> Subtract/1
  Subtract/1 -> Abslt_f32_f32/1
  Abslt_f32_f32/1 -> Relational Operator/1
  If/1 -> TrueOut_ResetRef/Action
  TrueOut_ResetRef/1(HwAgMoved) -> Merge/1
  FalseOut_KeepRef/1(HwAgMoved) -> Merge/2
  If/2 -> FalseOut_KeepRef/Action
  Merge/1 -> HwAgMoved/1
  FixdToFloat_f32_s16/1 -> Subtract/2

== system SF051A_SnsrOffsLrng/SnsrOffsLrng/SnsrOffsLrngPer1/EnableLearning/EnablingConditions/Subsystem5 ==

== system SF051A_SnsrOffsLrng/SnsrOffsLrng/SnsrOffsLrngPer1/EnableLearning/Eval_Time/GetTiSpan100MicroSec32bit ==
  note: Subtract original reference time
  note: seconds
  note: microseconds
  note: counts
  note: Wrap-to-zero
  note: 1 count = 100 uSec
  note: Get current system time
  note: GetTiSpan100MicroSec32bit
  note: Created Aug 18, 2015
      | Modified Oct 21, 2015
      | Modified Oct 30, 2015
      | Kevin Derry
  RefTmr : Inport
  CopyRight2 : Subsystem  Description=|  mask(Copyright Information){none=on}
      | Copyright info block.                                               
      |                                                                     
      | Place copyright information at the top of every subsystem in design.
      mask prompts: none "No parameters"
      mask help: Place copyright information at the top of every subsystem in design.
      mask Display:
      | NxtrConf = 'Nexteer Confidential';
      | 
      | sys = bdroot; %handle for the current model ("system")
      | first = get_param(sys,'Created');
      | if(isempty(first))
      |     first = datestr(now,'yyyy');
      | else
      |     first = first(end-3:end);  %year is last four digits
      | end
      | 
      | last = get_param(sys,'LastModifiedDate');
      | if isempty(last)
      |     last = datestr(now,'yyyy');
      | else
      |     last = last(end-3:end);
      | end
      | 
      | if strcmp(first,last)
      |     fprintf('%s -- Copyright %s Nexteer',NxtrConf,first)
      | else
      |     fprintf('%s -- %s%s- %s Nexteer',NxtrConf,char(169),first,last)
      | end
  Count per uSec : Constant  Value=0.01
  Data Store Read1 : DataStoreRead  DataStoreName=SimnTi
  Data Type Conversion2 : DataTypeConversion  OutDataTypeStr=uint32
  Divide1 : Product  Inputs=**
  Divide2 : Product  Inputs=*/
  If : If  NumInputs=2  IfExpression=u1 >= u2
  Max Counts : Constant  Value=2^32-1
  Merge : Merge
  No wrapping : Subsystem  TreatAsAtomicUnit=on
  Product2 : Product
  Product3 : Product
  Rounding : Rounding
  Subtract3 : Sum  Inputs=+-
  Wrapping : Subsystem  TreatAsAtomicUnit=on
  uSec per Sec : Constant  Value=1000000
  TiSpan : Outport
  wires:
  Wrapping/1(Out1) -> Merge/2
  No wrapping/1(Out1) -> Merge/1
  If/2 -> Wrapping/Action
  If/1 -> No wrapping/Action
  Product3/1 -> Subtract3/2
  Subtract3/1 -> Data Type Conversion2/1
  Rounding/1 -> Product3/1
  Divide2/1 -> Rounding/1
  Max Counts/1 -> Divide2/2, Product3/2
  Divide1/1 -> Divide2/1, Subtract3/1
  Product2/1 -> Divide1/1
  Data Store Read1/1 -> Product2/1
  Count per uSec/1 -> Divide1/2
  uSec per Sec/1 -> Product2/2
  Merge/1 -> TiSpan/1
  RefTmr/1 -> If/2, No wrapping/2(ref), Wrapping/2(ref)
  Data Type Conversion2/1 -> If/1, No wrapping/1(new), Wrapping/1(new)

== system SF051A_SnsrOffsLrng/SnsrOffsLrng/SnsrOffsLrngPer1/EnableLearning/Eval_Time/Subsystem5 ==

== system SF051A_SnsrOffsLrng/SnsrOffsLrng/SnsrOffsLrngPer1/EnableLearning/False_Reset/GetRefTmr100MicroSec32bit ==
  note: 1 count = 100 uSec
  note: seconds
  note: microseconds
  note: counts
  note: Wrap-to-zero
  note: GetRefTmr100MicroSec32bit
  note: Created Aug 18, 2015
      | Modified Oct 21, 2015
      | Modified Oct 30, 2015
      | Kevin Derry
  CopyRight2 : Subsystem  Description=|  mask(Copyright Information){none=on}
      | Copyright info block.                                               
      |                                                                     
      | Place copyright information at the top of every subsystem in design.
      mask prompts: none "No parameters"
      mask help: Place copyright information at the top of every subsystem in design.
      mask Display:
      | NxtrConf = 'Nexteer Confidential';
      | 
      | sys = bdroot; %handle for the current model ("system")
      | first = get_param(sys,'Created');
      | if(isempty(first))
      |     first = datestr(now,'yyyy');
      | else
      |     first = first(end-3:end);  %year is last four digits
      | end
      | 
      | last = get_param(sys,'LastModifiedDate');
      | if isempty(last)
      |     last = datestr(now,'yyyy');
      | else
      |     last = last(end-3:end);
      | end
      | 
      | if strcmp(first,last)
      |     fprintf('%s -- Copyright %s Nexteer',NxtrConf,first)
      | else
      |     fprintf('%s -- %s%s- %s Nexteer',NxtrConf,char(169),first,last)
      | end
  Count per uSec : Constant  Value=0.01
  Data Store Read1 : DataStoreRead  DataStoreName=SimnTi
  Data Type Conversion1 : DataTypeConversion  OutDataTypeStr=uint32
  Divide1 : Product  Inputs=**
  Divide2 : Product  Inputs=*/
  Max Counts : Constant  Value=2^32-1
  Product1 : Product
  Product2 : Product
  Rounding : Rounding
  Subtract1 : Sum  Inputs=+-
  uSec per Sec : Constant  Value=1000000
  RefTmr : Outport
  wires:
  Product2/1 -> Subtract1/2
  Subtract1/1 -> Data Type Conversion1/1
  Rounding/1 -> Product2/1
  Divide2/1 -> Rounding/1
  Max Counts/1 -> Divide2/2, Product2/2
  Divide1/1 -> Divide2/1, Subtract1/1
  Product1/1 -> Divide1/1
  Count per uSec/1 -> Divide1/2
  uSec per Sec/1 -> Product1/2
  Data Type Conversion1/1 -> RefTmr/1
  Data Store Read1/1 -> Product1/1

== system SF051A_SnsrOffsLrng/SnsrOffsLrng/SnsrOffsLrngPer1/EnableLearning/False_Reset/Subsystem5 ==

== system SF051A_SnsrOffsLrng/SnsrOffsLrng/SnsrOffsLrngPer1/EnableLearning/Filter_HwTq/Subsystem5 ==

== system SF051A_SnsrOffsLrng/SnsrOffsLrng/SnsrOffsLrngPer1/EnableLearning/Perform_TqInpDetn/Do nothing ==
  Action Port : ActionPort  ActionType=else
  Subsystem5 : Subsystem  Description=|  mask(Copyright Information){none=on}
      | Copyright info block.                                               
      |                                                                     
      | Place copyright information at the top of every subsystem in design.
      mask prompts: none "No parameters"
      mask help: Place copyright information at the top of every subsystem in design.
      mask Display:
      | NxtrConf = 'Nexteer Confidential';
      | 
      | sys = bdroot; %handle for the current model ("system")
      | first = get_param(sys,'Created');
      | first = first(end-3:end);  %year is last four digits
      | 
      | last = get_param(sys,'LastModifiedDate');
      | if isempty(last)
      |     last = datestr(now,'yyyy');
      | else
      |     last = last(end-3:end);
      | end
      | 
      | if strcmp(first,last)
      |     fprintf('%s -- Copyright %s Nexteer',NxtrConf,first)
      | else
      |     fprintf('%s -- %s%s- %s Nexteer',NxtrConf,char(169),first,last)
      | end

== system SF051A_SnsrOffsLrng/SnsrOffsLrng/SnsrOffsLrngPer1/EnableLearning/Perform_TqInpDetn/ElapsedTime ==
  note: Limit changed to a Min block.
  Add : Sum
  Data Store Read : DataStoreRead  DataStoreName=TqInpDetnEnaTi
  Data Store Write : DataStoreWrite  DataStoreName=TqInpDetnEnaTi
  Min_f32 : NxtrMin/Min_f32  SFunctionSpec=single y1 = Min_f32(single u1, single u2)
      settings: AttributesFormatString=%<Name>
  Subsystem5 : Subsystem  Description=|  mask(Copyright Information){none=on}
      | Copyright info block.                                               
      |                                                                     
      | Place copyright information at the top of every subsystem in design.
      mask prompts: none "No parameters"
      mask help: Place copyright information at the top of every subsystem in design.
      mask Display:
      | NxtrConf = 'Nexteer Confidential';
      | 
      | sys = bdroot; %handle for the current model ("system")
      | first = get_param(sys,'Created');
      | first = first(end-3:end);  %year is last four digits
      | 
      | last = get_param(sys,'LastModifiedDate');
      | if isempty(last)
      |     last = datestr(now,'yyyy');
      | else
      |     last = last(end-3:end);
      | end
      | 
      | if strcmp(first,last)
      |     fprintf('%s -- Copyright %s Nexteer',NxtrConf,first)
      | else
      |     fprintf('%s -- %s%s- %s Nexteer',NxtrConf,char(169),first,last)
      | end
  Ts : Constant  Value=ARCHGLBPRM_2MILLISEC_SEC_F32
  Ts1 : Constant  Value=HWTQLRNGTMRHILIM_SEC_F32
  TiEnad : Outport
  wires:
  Ts/1 -> Add/1
  Data Store Read/1 -> Add/2
  Add/1 -> Min_f32/1
  Min_f32/1 -> Data Store Write/1, TiEnad/1
  Ts1/1 -> Min_f32/2

== system SF051A_SnsrOffsLrng/SnsrOffsLrng/SnsrOffsLrngPer1/EnableLearning/Perform_TqInpDetn/Enable_PreProcessing ==
  note: Logic was reordered to avoid coverage issues. No functional change
  note: Enable_PreProcessing == true
  TiEnad : Inport
  HwTqFild : Inport  Port=2
  Constant : Constant  Value=SnsrOffsLrngTqInpDetnPwrEstimnThd
  Constant2 : Constant  Value=ARCHGLBPRM_2MILLISEC_SEC_F32
  Display : DataStoreWrite  DataStoreName=dSnsrOffsLrngTqInpPrsntRaw
  False_Hold : Subsystem  TreatAsAtomicUnit=on
  If Action Subsystem : Subsystem  TreatAsAtomicUnit=on
  If1 : If  IfExpression=u1
  Merge_Present : Merge
  Merge_Validity : Merge
  Preprocessing : Subsystem
  Product : Product
  Relational Operator : RelationalOperator  OutDataTypeStr=boolean
  Relational Operator1 : RelationalOperator  Operator=>  OutDataTypeStr=boolean
  Subsystem5 : Subsystem  Description=|  mask(Copyright Information){none=on}
      | Copyright info block.                                               
      |                                                                     
      | Place copyright information at the top of every subsystem in design.
      mask prompts: none "No parameters"
      mask help: Place copyright information at the top of every subsystem in design.
      mask Display:
      | NxtrConf = 'Nexteer Confidential';
      | 
      | sys = bdroot; %handle for the current model ("system")
      | first = get_param(sys,'Created');
      | first = first(end-3:end);  %year is last four digits
      | 
      | last = get_param(sys,'LastModifiedDate');
      | if isempty(last)
      |     last = datestr(now,'yyyy');
      | else
      |     last = last(end-3:end);
      | end
      | 
      | if strcmp(first,last)
      |     fprintf('%s -- Copyright %s Nexteer',NxtrConf,first)
      | else
      |     fprintf('%s -- %s%s- %s Nexteer',NxtrConf,char(169),first,last)
      | end
  TqInpPrsntVld : Outport  InitialOutput=0
  TqInpPrsnt : Outport  Port=2  InitialOutput=0
  wires:
  Preprocessing/2(HwTrqPreproc) -> Relational Operator1/1
  HwTqFild/1 -> Preprocessing/1(HwTqFild)
  Product/1 -> Relational Operator/2  "TqInpDetnBufTi"
  TiEnad/1 -> Relational Operator/1
  Relational Operator/1 -> If1/1  "HwTqPreprocVld"
  Constant/1 -> Relational Operator1/2
  Relational Operator1/1 -> If Action Subsystem/1(TqInpPrsntRaw), Display/1  "TqInpPrsntRaw"
  If Action Subsystem/1(TqInpPrsntVld) -> Merge_Validity/1
  False_Hold/1(Vld) -> Merge_Validity/2
  Merge_Validity/1 -> TqInpPrsntVld/1
  If Action Subsystem/2(TqInpPrsnt) -> Merge_Present/1
  False_Hold/2(Prsnt) -> Merge_Present/2
  Merge_Present/1 -> TqInpPrsnt/1
  Preprocessing/1(SampleCntrLim) -> Product/2
  Constant2/1 -> Product/1
  If1/2 -> False_Hold/Action
  If1/1 -> If Action Subsystem/Action
